simulink model "AION_auto_mode_request"  (R2021a)
settings: configuration reference "AION_IDS_Speedgoat" (kept outside this file)
settings Model: DataDictionary=AION_auto_mode_request.sldd  SimulationMode=external  Creator=Administrator  LastModifiedBy=Administrator
settings ConfigSetRef: SourceName=AION_IDS_Speedgoat

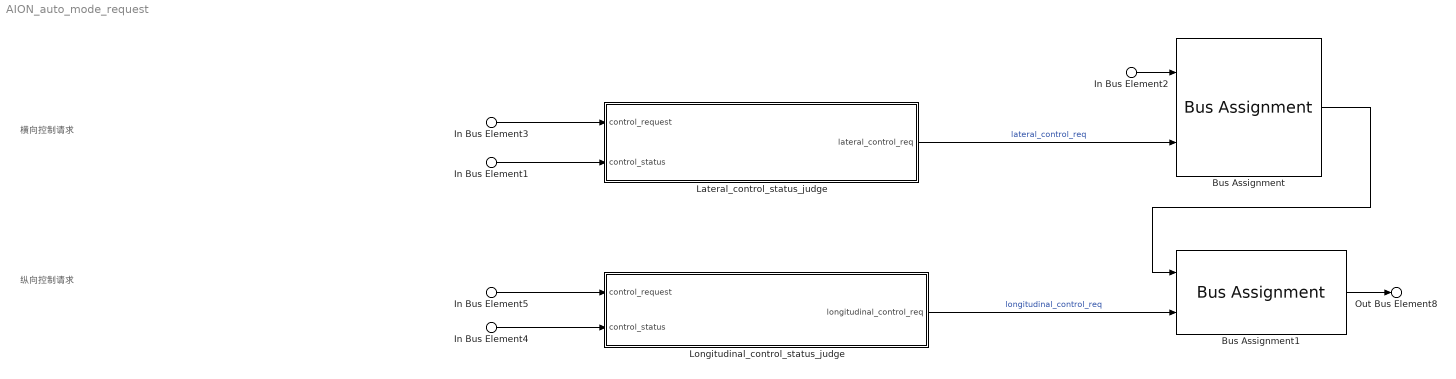
== system AION_auto_mode_request ==
  note: 横向控制请求
  note: 纵向控制请求
  In Bus Element2 : Inport  PortName=InBus
  In Bus Element3 : Inport  PortName=InBus  Element=set_lateral_control_info.set_LatCtrlReq
  In Bus Element5 : Inport  PortName=InBus  Element=set_longitudinal_control_info.set_LngCtrlReq
  In Bus Element1 : Inport  PortName=InBus  Element=get_SCU_info.get_LatCtrlMode
  In Bus Element4 : Inport  PortName=InBus  Element=get_SCU_info.get_LngCtrlMode
  Bus Assignment : BusAssignment  AssignedSignals=set_lateral_control_info.set_LatCtrlReq
  Bus Assignment1 : BusAssignment  AssignedSignals=set_longitudinal_control_info.set_LngCtrlReq
  Lateral_control_status_judge : MATLAB Function  TreatAsAtomicUnit=on
  Longitudinal_control_status_judge : MATLAB Function  TreatAsAtomicUnit=on
  Out Bus Element8 : Outport  PortName=OutBus
  wires:
  Lateral_control_status_judge/1(lateral_control_req) -> Bus Assignment/2  "lateral_control_req"
  In Bus Element2/1 -> Bus Assignment/1
  Bus Assignment/1 -> Bus Assignment1/1
  In Bus Element4/1 -> Longitudinal_control_status_judge/2(control_status)
  Longitudinal_control_status_judge/1(longitudinal_control_req) -> Bus Assignment1/2  "longitudinal_control_req"
  In Bus Element3/1 -> Lateral_control_status_judge/1(control_request)
  In Bus Element5/1 -> Longitudinal_control_status_judge/1(control_request)
  In Bus Element1/1 -> Lateral_control_status_judge/2(control_status)
  Bus Assignment1/1 -> Out Bus Element8/1

== matlab function AION_auto_mode_request/Longitudinal_control_status_judge ==
  data: control_request input; control_status input Enum: Control_status size=1; longitudinal_control_req output Enum: Control_request size=1
% 操作模式判断
function longitudinal_control_req = longitudinal_control_status_judge(control_request,control_status)
%   1.输入参数：
%       (1)control_request           纵向控制请求的实际值
%       (2)control_status            纵向控制功能状态
        
%   2.输出参数：
%       (1)longitudinal_control_req       纵向控制请求的期望值

%%
if(control_request == Control_request.Auto)
    %车辆上电过程，使车辆进入自动控制状态
    switch control_status 
        case Control_status.QuitStatus
        longitudinal_control_req = Control_request.Manual;
        case Control_status.ManualStatus
        longitudinal_control_req = Control_request.Auto;
         case Control_status.AutoStatus
        longitudinal_control_req = Control_request.Auto;
        otherwise
        longitudinal_control_req = Control_request.Manual;
    end
else
    longitudinal_control_req = Control_request.Manual;
end
end

== matlab function AION_auto_mode_request/Lateral_control_status_judge ==
  data: control_request input; control_status input Enum: Control_status size=1; lateral_control_req output Enum: Control_request size=1
% 操作模式判断
function lateral_control_req = lateral_control_status_judge(control_request,control_status)
%   1.输入参数：
%       (1)control_status            横向控制功能状态
%   2.输出参数：
%       (1)lateral_control_req       横向控制请求

%%

if(control_request == Control_request.Auto)
%     车辆上电过程，使车辆进入自动控制状态
    switch control_status 
        case Control_status.QuitStatus
        lateral_control_req = Control_request.Manual;
        case Control_status.ManualStatus
        lateral_control_req = Control_request.Auto;
        case Control_status.AutoStatus
        lateral_control_req = Control_request.Auto;
        otherwise %Fault_status
        lateral_control_req = Control_request.Manual;
    end
else
    lateral_control_req = Control_request.Manual;
end

% lateral_control_req = Control_request.Manual;
end
